simulink model "trans_fail_demo"  (R2021a)
settings: Solver=FixedStepAuto  StartTime=0.0  StopTime=10.0  FixedStep=0.1  RelTol=1e-3
settings Model: Creator=DELL  LastModifiedBy=DELL

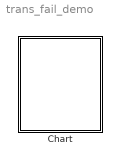
== system trans_fail_demo ==
  Chart : Stateflow chart  TreatAsAtomicUnit=on

== stateflow chart trans_fail_demo/Chart ==
  state ddd [parallel]
    en:
    res = 0;
    du:
    sfdbg('ddd.du')
    on every(5, tick):
    res= 0;
    send(E, ddd1)
    if (in(ddd1.b))
    sfdbg('tr success  in')
    else
    sfdbg('tr.failed in')
    end
    if (res ==1)
    sfdbg('tr success')
    else
    sfdbg('tr.failed')
    end
    settings: executionOrder=1
  state ddd1 [parallel]
    settings: executionOrder=2
    state a
      on E:
      sfdbg('a tran failed')
    state b
      en:
      sfdbg('a trans succed')
    (default) -> b
    a -> b : E[getSimulationTime>1.2]/{res=1;}
    b -> a : E/{res=1;}
  data: res local
  events: E local FUNCTION_CALL_EVENT
